simulink model "QEI_READ"  (R2024b)
settings: Solver=FixedStepAuto  StartTime=0.0  StopTime=inf  FixedStep=0.1  RelTol=1e-3  EnableMultiTasking=on
libraries: stm32f4xxblockslib x8, stm32g4xxblockslib x6, simulink x4
settings Model: STM32="{\"EncoderBlockForG4\":[{\"ID\":\"QEI_READ:1\"},{\"ID\":\"QEI_READ:14\"},{\"ID\":\"QEI_READ:15\"},{\"ID\":\"QEI_READ:106\"},{\"ID\":\"QEI_READ:107\"},{\"ID\":\"QEI_READ:108\"}],\"DigitalPortRead\":[{\"ID\":\"QEI_READ:3\"},{\"ID\":\"QEI_READ:4\"},{\"ID\":\"QEI_READ:55\"},{\"ID\":\"QEI_READ:64\"},{\"ID\":\"QEI_READ:78\"},{\"ID\":\"QEI_READ:79\"},{\"ID\":\"QEI_READ:80\"},{\"ID\":\"QEI_READ:81\"}]}"  Creator=asus  LastModifiedBy=asus
settings OptimizationCC: DefaultParameterBehavior=Inlined  EnhancedBackFolding=on  PassReuseOutputArgsAs=Individual arguments  ZeroExternalMemoryAtStartup=off  ZeroInternalMemoryAtStartup=off  MaxStackSize=512  OptimizeBlockOrder=speed  DifferentSizesBufferReuse=on  OptimizationCustomize=off  EfficientTunableParamExpr=on
settings DebuggingCC: ParameterTunabilityLossMsg=error
settings HardwareCC: ProdBitPerPointer=32  ProdBitPerSizeT=32  ProdBitPerPtrDiffT=32  ProdLargestAtomicInteger=Long  ProdLargestAtomicFloat=Double  ProdWordSize=32  ProdLongLongMode=on  ProdHWDeviceType=ARM Compatible->ARM Cortex-M
settings SFSimCC: MATLABDynamicMemAlloc=off
settings RTWCC: Description=Embedded Coder  SystemTargetFile=ert.tlc  HardwareBoard=STM32G4xx Based  TemplateMakefile=ert_default_tmf  Toolchain=GNU Tools for ARM Embedded Processors
settings CodeAppCC: ForceParamTrailComments=on  IgnoreCustomStorageClasses=off  OperatorAnnotations=on  SimulinkDataObjDesc=on  SFDataObjDesc=on  InsertBlockDesc=on
settings ERTTargetCC: TargetLangStandard=C99 (ISO)  CodeReplacementLibrary=ARM Cortex-M  ExtModeTransport=3  ExtModeStaticAlloc=on  ExtModeStaticAllocSize=2048  ExtModeMexFile=ext_xcp  ExtModeIntrfLevel=Level2 - Open

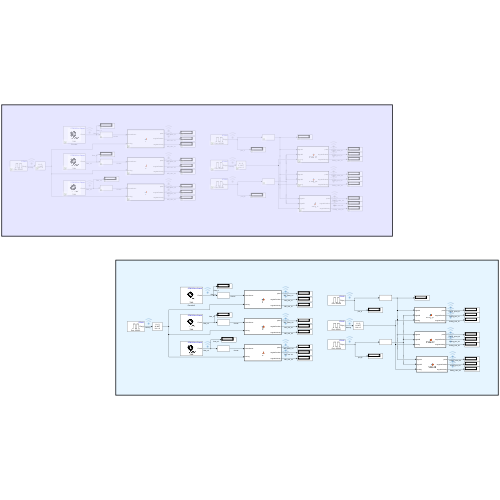
[thumbnail: Simulink's stored preview of the top-level diagram]
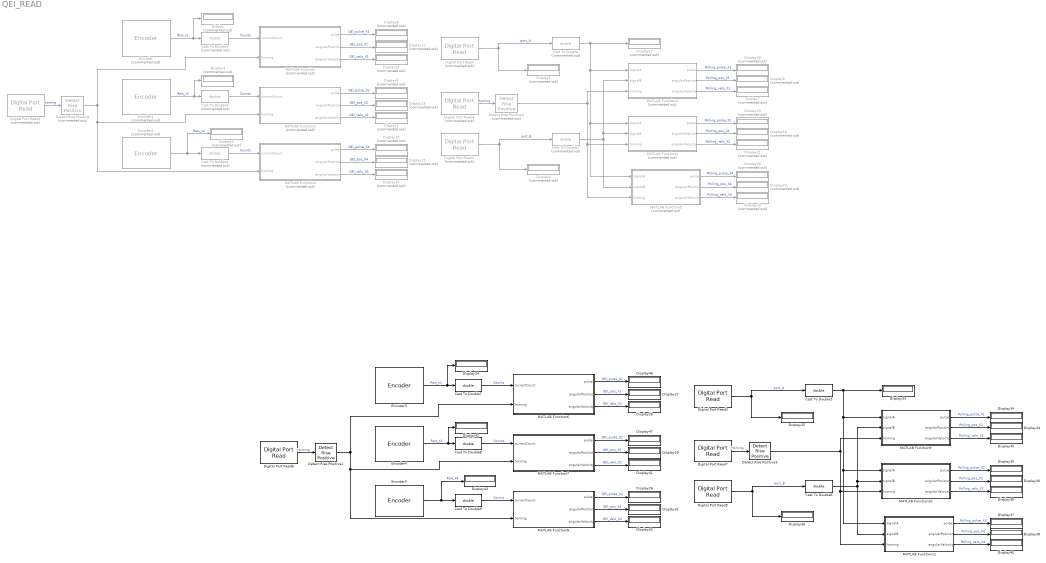
== system QEI_READ ==
  Cast To Double{,1..4} (5 alike) : DataTypeConversion  Commented=on  OutDataTypeStr=double  SaturateOnIntegerOverflow=off  RndMeth=Floor
  Cast To Double{5..9} (5 alike) : DataTypeConversion  OutDataTypeStr=double  SaturateOnIntegerOverflow=off  RndMeth=Floor
  Detect Rise Positive : simulink/Logic and Bit Operations/Detect Rise Positive  Commented=on  vinit=0  OutDataTypeStr=boolean
  Detect Rise Positive1 : simulink/Logic and Bit Operations/Detect Rise Positive  vinit=0  OutDataTypeStr=boolean
  Detect Rise Positive2 : simulink/Logic and Bit Operations/Detect Rise Positive  Commented=on  vinit=0  OutDataTypeStr=boolean
  Detect Rise Positive3 : simulink/Logic and Bit Operations/Detect Rise Positive  vinit=0  OutDataTypeStr=boolean
  Digital Port Read : stm32f4xxblockslib/Digital Port Read  Commented=on  PortName=GPIOB  PinNumber=[10]  ReadOperation=on  IOAsArray=on  SampleTime=-1  EnableSimPort=off  hoistedMaskSrc=ECSoC/ECSimCodegen/Digital Port Read
      settings: LibrarySourceBlock=stm32g4xxblockslib/Digital Port Read
  Digital Port Read1 : stm32f4xxblockslib/Digital Port Read  Commented=on  PortName=GPIOB  PinNumber=[4]  ReadOperation=on  IOAsArray=on  SampleTime=-1  EnableSimPort=off  hoistedMaskSrc=ECSoC/ECSimCodegen/Digital Port Read
      settings: LibrarySourceBlock=stm32g4xxblockslib/Digital Port Read
  Digital Port Read2 : stm32f4xxblockslib/Digital Port Read  Commented=on  PortName=GPIOC  PinNumber=[13]  ReadOperation=on  IOAsArray=on  SampleTime=-1  EnableSimPort=off  hoistedMaskSrc=ECSoC/ECSimCodegen/Digital Port Read
      settings: LibrarySourceBlock=stm32g4xxblockslib/Digital Port Read
  Digital Port Read3 : stm32f4xxblockslib/Digital Port Read  PortName=GPIOB  PinNumber=[10]  ReadOperation=on  IOAsArray=on  SampleTime=-1  EnableSimPort=off  hoistedMaskSrc=ECSoC/ECSimCodegen/Digital Port Read
      settings: LibrarySourceBlock=stm32g4xxblockslib/Digital Port Read
  Digital Port Read4 : stm32f4xxblockslib/Digital Port Read  Commented=on  PortName=GPIOC  PinNumber=[13]  ReadOperation=on  IOAsArray=on  SampleTime=-1  EnableSimPort=off  hoistedMaskSrc=ECSoC/ECSimCodegen/Digital Port Read
      settings: LibrarySourceBlock=stm32g4xxblockslib/Digital Port Read
  Digital Port Read5 : stm32f4xxblockslib/Digital Port Read  PortName=GPIOB  PinNumber=[4]  ReadOperation=on  IOAsArray=on  SampleTime=-1  EnableSimPort=off  hoistedMaskSrc=ECSoC/ECSimCodegen/Digital Port Read
      settings: LibrarySourceBlock=stm32g4xxblockslib/Digital Port Read
  Digital Port Read6 : stm32f4xxblockslib/Digital Port Read  PortName=GPIOC  PinNumber=[13]  ReadOperation=on  IOAsArray=on  SampleTime=-1  EnableSimPort=off  hoistedMaskSrc=ECSoC/ECSimCodegen/Digital Port Read
      settings: LibrarySourceBlock=stm32g4xxblockslib/Digital Port Read
  Digital Port Read7 : stm32f4xxblockslib/Digital Port Read  PortName=GPIOC  PinNumber=[13]  ReadOperation=on  IOAsArray=on  SampleTime=-1  EnableSimPort=off  hoistedMaskSrc=ECSoC/ECSimCodegen/Digital Port Read
      settings: LibrarySourceBlock=stm32g4xxblockslib/Digital Port Read
  Display{,1..23} (24 alike) : Display  Commented=on
  Display{24..47} (24 alike) : Display
  Encoder : stm32g4xxblockslib/Encoder  Commented=on  TimerModule=TIM3  EnableResetInput=off  OutputCountAfterFirstIndex=off  OutputValidIndex=off  OutputDirection=off  OutputStatus=off  SampleTime=-1
  Encoder1 : stm32g4xxblockslib/Encoder  Commented=on  TimerModule=TIM4  EnableResetInput=off  OutputCountAfterFirstIndex=off  OutputValidIndex=off  OutputDirection=off  OutputStatus=off  SampleTime=-1
  Encoder2 : stm32g4xxblockslib/Encoder  Commented=on  TimerModule=TIM8  EnableResetInput=off  OutputCountAfterFirstIndex=off  OutputValidIndex=off  OutputDirection=off  OutputStatus=off  SampleTime=-1
  Encoder3 : stm32g4xxblockslib/Encoder  TimerModule=TIM3  EnableResetInput=off  OutputCountAfterFirstIndex=off  OutputValidIndex=off  OutputDirection=off  OutputStatus=off  SampleTime=-1
  Encoder4 : stm32g4xxblockslib/Encoder  TimerModule=TIM4  EnableResetInput=off  OutputCountAfterFirstIndex=off  OutputValidIndex=off  OutputDirection=off  OutputStatus=off  SampleTime=-1
  Encoder5 : stm32g4xxblockslib/Encoder  TimerModule=TIM8  EnableResetInput=off  OutputCountAfterFirstIndex=off  OutputValidIndex=off  OutputDirection=off  OutputStatus=off  SampleTime=-1
  MATLAB Function : MATLAB Function  Commented=on  TreatAsAtomicUnit=on
  MATLAB Function1 : MATLAB Function  Commented=on  TreatAsAtomicUnit=on
  MATLAB Function10 : MATLAB Function  TreatAsAtomicUnit=on
  MATLAB Function11 : MATLAB Function  TreatAsAtomicUnit=on
  MATLAB Function2 : MATLAB Function  Commented=on  TreatAsAtomicUnit=on
  MATLAB Function3 : MATLAB Function  Commented=on  TreatAsAtomicUnit=on
  MATLAB Function4 : MATLAB Function  Commented=on  TreatAsAtomicUnit=on
  MATLAB Function5 : MATLAB Function  Commented=on  TreatAsAtomicUnit=on
  MATLAB Function6 : MATLAB Function  TreatAsAtomicUnit=on
  MATLAB Function7 : MATLAB Function  TreatAsAtomicUnit=on
  MATLAB Function8 : MATLAB Function  TreatAsAtomicUnit=on
  MATLAB Function9 : MATLAB Function  TreatAsAtomicUnit=on
  wires:
  Encoder/1 -> Display/1, Cast To Double2/1  "Raw_x1"
  Digital Port Read/1 -> Cast To Double/1, Display1/1  "port_A"
  Digital Port Read1/1 -> Cast To Double1/1, Display2/1  "port_B"
  Cast To Double2/1 -> MATLAB Function/1(currentCount)  "Counts"
  MATLAB Function/1(pulse) -> Display8/1  "QEI_pulse_X1"
  MATLAB Function1/1(pulse) -> Display9/1  "QEI_pulse_X2"
  Cast To Double3/1 -> MATLAB Function1/1(currentCount)  "Counts"
  Cast To Double4/1 -> MATLAB Function2/1(currentCount)  "Counts"
  MATLAB Function2/1(pulse) -> Display10/1  "QEI_pulse_X4"
  MATLAB Function/2(angularPosition) -> Display11/1  "QEI_pos_X1"
  MATLAB Function1/2(angularPosition) -> Display13/1  "QEI_pos_X2"
  MATLAB Function2/2(angularPosition) -> Display15/1  "QEI_pos_X4"
  MATLAB Function2/3(angularVelocity) -> Display16/1  "QEI_velo_X4"
  Cast To Double/1 -> Display17/1, MATLAB Function5/1(signalA), MATLAB Function4/1(signalA), MATLAB Function3/1(signalA)
  MATLAB Function3/1(pulse) -> Display18/1  "Polling_pulse_X1"
  MATLAB Function4/1(pulse) -> Display19/1  "Polling_pulse_X2"
  MATLAB Function5/1(pulse) -> Display20/1  "Polling_pulse_X4"
  Cast To Double1/1 -> MATLAB Function4/2(signalB), MATLAB Function3/2(signalB), MATLAB Function5/2(signalB)
  MATLAB Function1/3(angularVelocity) -> Display3/1  "QEI_velo_X2"
  MATLAB Function/3(angularVelocity) -> Display12/1  "QEI_velo_X1"
  Digital Port Read2/1 -> Detect Rise Positive/1  "Homing"
  Detect Rise Positive/1 -> MATLAB Function2/2(homing), MATLAB Function1/2(homing), MATLAB Function/2(homing)
  Encoder1/1 -> Display4/1, Cast To Double3/1  "Raw_x2"
  Encoder2/1 -> Display5/1, Cast To Double4/1  "Raw_x4"
  Digital Port Read4/1 -> Detect Rise Positive2/1  "Homing"
  Detect Rise Positive2/1 -> MATLAB Function5/3(homing), MATLAB Function4/3(homing), MATLAB Function3/3(homing)
  MATLAB Function3/2(angularPosition) -> Display6/1  "Polling_pos_X1"
  MATLAB Function3/3(angularVelocity) -> Display7/1  "Polling_velo_X1"
  MATLAB Function4/2(angularPosition) -> Display14/1  "Polling_pos_X2"
  MATLAB Function4/3(angularVelocity) -> Display21/1  "Polling_velo_X2"
  MATLAB Function5/2(angularPosition) -> Display22/1  "Polling_pos_X4"
  MATLAB Function5/3(angularVelocity) -> Display23/1  "Polling_velo_X4"
  MATLAB Function6/1(pulse) -> Display46/1  "QEI_pulse_X1"
  MATLAB Function7/3(angularVelocity) -> Display41/1  "QEI_velo_X2"
  Digital Port Read5/1 -> Cast To Double6/1, Display36/1  "port_B"
  Cast To Double7/1 -> MATLAB Function6/1(currentCount)  "Counts"
  Digital Port Read6/1 -> Detect Rise Positive1/1  "Homing"
  MATLAB Function7/2(angularPosition) -> Display29/1  "QEI_pos_X2"
  Detect Rise Positive1/1 -> MATLAB Function8/2(homing), MATLAB Function7/2(homing), MATLAB Function6/2(homing)
  Encoder5/1 -> Display43/1, Cast To Double9/1  "Raw_x4"
  Cast To Double6/1 -> MATLAB Function10/2(signalB), MATLAB Function9/2(signalB), MATLAB Function11/2(signalB)
  MATLAB Function9/1(pulse) -> Display34/1  "Polling_pulse_X1"
  MATLAB Function10/3(angularVelocity) -> Display38/1  "Polling_velo_X2"
  MATLAB Function9/3(angularVelocity) -> Display45/1  "Polling_velo_X1"
  MATLAB Function6/2(angularPosition) -> Display27/1  "QEI_pos_X1"
  Digital Port Read3/1 -> Cast To Double5/1, Display25/1  "port_A"
  MATLAB Function8/1(pulse) -> Display26/1  "QEI_pulse_X4"
  Cast To Double5/1 -> Display33/1, MATLAB Function11/1(signalA), MATLAB Function10/1(signalA), MATLAB Function9/1(signalA)
  MATLAB Function9/2(angularPosition) -> Display44/1  "Polling_pos_X1"
  Cast To Double8/1 -> MATLAB Function7/1(currentCount)  "Counts"
  Digital Port Read7/1 -> Detect Rise Positive3/1  "Homing"
  MATLAB Function8/2(angularPosition) -> Display31/1  "QEI_pos_X4"
  Detect Rise Positive3/1 -> MATLAB Function11/3(homing), MATLAB Function10/3(homing), MATLAB Function9/3(homing)
  MATLAB Function11/2(angularPosition) -> Display39/1  "Polling_pos_X4"
  MATLAB Function6/3(angularVelocity) -> Display28/1  "QEI_velo_X1"
  MATLAB Function10/1(pulse) -> Display35/1  "Polling_pulse_X2"
  Encoder3/1 -> Display24/1, Cast To Double7/1  "Raw_x1"
  MATLAB Function11/3(angularVelocity) -> Display40/1  "Polling_velo_X4"
  MATLAB Function7/1(pulse) -> Display47/1  "QEI_pulse_X2"
  MATLAB Function11/1(pulse) -> Display37/1  "Polling_pulse_X4"
  MATLAB Function8/3(angularVelocity) -> Display32/1  "QEI_velo_X4"
  Encoder4/1 -> Display42/1, Cast To Double8/1  "Raw_x2"
  Cast To Double9/1 -> MATLAB Function8/1(currentCount)  "Counts"
  MATLAB Function10/2(angularPosition) -> Display30/1  "Polling_pos_X2"

== matlab function QEI_READ/MATLAB Function6 ==
  data: pulse output; currentCount input; angularPosition output; angularVelocity output; homing input
function [pulse, angularPosition, angularVelocity] = X1(currentCount, homing)
    % พารามิเตอร์ที่ใช้ในการคำนวณ
    maxCount = 65534;           % ค่าสูงสุดที่สามารถนับได้ก่อนจะ wrap-around
    timeInterval = 0.1;         % ช่วงเวลาที่ใช้ในการคำนวณความเร็วเชิงมุม (วินาที)
    PPR = 2048;                   % จำนวนพัลส์ต่อรอบของ Encoder (Pulses Per Revolution)

    % Persistent Variables เพื่อเก็บค่าก่อนหน้า
    persistent previousCount totalCount previousRadians homepos

    % ตั้งค่าเริ่มต้นสำหรับ Persistent Variables
    if isempty(previousCount)
        previousCount = currentCount;
        totalCount = 0;
        previousRadians = 0;
        homepos = 0;
    end

    % คำนวณความแตกต่างระหว่าง currentCount และ previousCount
    diffCount = currentCount - previousCount;

    % ตรวจสอบการเกิด wrap-around
    if diffCount < -maxCount/2
        totalCount = totalCount + (maxCount + diffCount);  % Wrap-around จาก maxCount กลับไปที่ 0
    elseif diffCount > maxCount/2
        totalCount = totalCount + (diffCount - maxCount);  % Wrap-around จาก 0 ไปที่ maxCount
    else
        totalCount = totalCount + diffCount;               % กรณีปกติ ไม่มีการ wrap-around
    end

    % ตั้งค่าโฮม (Home Position) เมื่อ homing == 1
    if homing == 1
        homepos = totalCount;
    end

    % คำนวณตำแหน่งเชิงมุม (Angular Position) และความเร็วเชิงมุม (Angular Velocity)
    pulse = totalCount - homepos;                             % จำนวนพัลส์นับจากตำแหน่งโฮม
    angularPosition = (pulse / PPR) * 2 * pi;                 % แปลงจำนวนพัลส์เป็นตำแหน่งเชิงมุม (radians)
    angularVelocity = (angularPosition - previousRadians) / timeInterval;  % คำนวณความเร็วเชิงมุม

    % อัปเดตค่าก่อนหน้า
    previousCount = currentCount;
    previousRadians = angularPosition;
end

== matlab function QEI_READ/MATLAB Function7 ==
  data: pulse output; currentCount input; angularPosition output; angularVelocity output; homing input
function [pulse, angularPosition, angularVelocity] = X2(currentCount, homing)
    % พารามิเตอร์ที่ใช้ในการคำนวณ
    maxCount = 65534;           % ค่าสูงสุดที่สามารถนับได้ก่อนจะ wrap-around
    timeInterval = 0.1;         % ช่วงเวลาที่ใช้ในการคำนวณความเร็วเชิงมุม (วินาที)
    PPR = 2048;                   % จำนวนพัลส์ต่อรอบของ Encoder (Pulses Per Revolution)

    % Persistent Variables เพื่อเก็บค่าก่อนหน้า
    persistent previousCount totalCount previousRadians homepos

    % ตั้งค่าเริ่มต้นสำหรับ Persistent Variables
    if isempty(previousCount)
        previousCount = currentCount;
        totalCount = 0;
        previousRadians = 0;
        homepos = 0;
    end

    % คำนวณความแตกต่างระหว่าง currentCount และ previousCount
    diffCount = currentCount - previousCount;

    % ตรวจสอบการเกิด wrap-around
    if diffCount < -maxCount/2
        totalCount = totalCount + (maxCount + diffCount);  % Wrap-around จาก maxCount กลับไปที่ 0
    elseif diffCount > maxCount/2
        totalCount = totalCount + (diffCount - maxCount);  % Wrap-around จาก 0 ไปที่ maxCount
    else
        totalCount = totalCount + diffCount;               % กรณีปกติ ไม่มีการ wrap-around
    end

    % ตั้งค่าโฮม (Home Position) เมื่อ homing == 1
    if homing == 1
        homepos = totalCount;
    end

    % คำนวณตำแหน่งเชิงมุม (Angular Position) และความเร็วเชิงมุม (Angular Velocity)
    pulse = totalCount - homepos;                             % จำนวนพัลส์นับจากตำแหน่งโฮม
    angularPosition = (pulse / PPR) * 2 * pi;                 % แปลงจำนวนพัลส์เป็นตำแหน่งเชิงมุม (radians)
    angularVelocity = (angularPosition - previousRadians) / timeInterval;  % คำนวณความเร็วเชิงมุม

    % อัปเดตค่าก่อนหน้า
    previousCount = currentCount;
    previousRadians = angularPosition;
end

== matlab function QEI_READ/MATLAB Function8 ==
  data: pulse output; currentCount input; angularPosition output; angularVelocity output; homing input
function [pulse, angularPosition, angularVelocity] = X4(currentCount, homing)
    % พารามิเตอร์ที่ใช้ในการคำนวณ
    % พารามิเตอร์ที่ใช้ในการคำนวณ
    maxCount = 65534;           % ค่าสูงสุดที่สามารถนับได้ก่อนจะ wrap-around
    timeInterval = 0.1;         % ช่วงเวลาที่ใช้ในการคำนวณความเร็วเชิงมุม (วินาที)
    PPR = 2048;                   % จำนวนพัลส์ต่อรอบของ Encoder (Pulses Per Revolution)

    % Persistent Variables เพื่อเก็บค่าก่อนหน้า
    persistent previousCount totalCount previousRadians homepos

    % ตั้งค่าเริ่มต้นสำหรับ Persistent Variables
    if isempty(previousCount)
        previousCount = currentCount;
        totalCount = 0;
        previousRadians = 0;
        homepos = 0;
    end

    % คำนวณความแตกต่างระหว่าง currentCount และ previousCount
    diffCount = currentCount - previousCount;

    % ตรวจสอบการเกิด wrap-around
    if diffCount < -maxCount/2
        totalCount = totalCount + (maxCount + diffCount);  % Wrap-around จาก maxCount กลับไปที่ 0
    elseif diffCount > maxCount/2
        totalCount = totalCount + (diffCount - maxCount);  % Wrap-around จาก 0 ไปที่ maxCount
    else
        totalCount = totalCount + diffCount;               % กรณีปกติ ไม่มีการ wrap-around
    end

    % ตั้งค่าโฮม (Home Position) เมื่อ homing == 1
    if homing == 1
        homepos = totalCount;
    end

    % คำนวณตำแหน่งเชิงมุม (Angular Position) และความเร็วเชิงมุม (Angular Velocity)
    pulse = totalCount - homepos;                             % จำนวนพัลส์นับจากตำแหน่งโฮม
    angularPosition = (pulse / PPR) * 2 * pi;                 % แปลงจำนวนพัลส์เป็นตำแหน่งเชิงมุม (radians)
    angularVelocity = (angularPosition - previousRadians) / timeInterval;  % คำนวณความเร็วเชิงมุม

    % อัปเดตค่าก่อนหน้า
    previousCount = currentCount;
    previousRadians = angularPosition;
end

== matlab function QEI_READ/MATLAB Function9 ==
  data: signalA input; pulse output; signalB input; homing input; angularPosition output; angularVelocity output
function [pulse, angularPosition, angularVelocity] = Polling_X1(signalA, signalB, homing)
    % กำหนดค่าพารามิเตอร์
    PPR = 2048;               % จำนวนพัลส์ต่อรอบ
    timeInterval = 0.1;     % ช่วงเวลาที่ใช้ในการคำนวณความเร็วเชิงมุม

    % ตัวแปร persistent เพื่อเก็บค่าก่อนหน้าและจำนวนพัลส์ต่อเนื่อง
    persistent previousCount totalCount homepos previousRadians

    % กำหนดค่าเริ่มต้นเมื่อฟังก์ชันถูกเรียกครั้งแรก
    if isempty(previousCount)
        previousCount = 0;
        totalCount = 0;
        homepos = 0;
        previousRadians = 0;
    end

    % คำนวณจำนวนพัลส์ต่อเนื่องตามสัญญาณ A และ B
    if signalA == 1 && signalB == 0
        totalCount = previousCount + 1; % หมุนในทิศทางตามเข็มนาฬิกา
    elseif signalA == 0 && signalB == 1
        totalCount = previousCount - 1; % หมุนในทิศทางตรงกันข้าม
    else
        totalCount = previousCount; % ไม่มีการเปลี่ยนแปลง
    end

% กำหนดตำแหน่งเริ่มต้น (home position) หากอยู่ในโหมด homing
    if homing == 1
        homepos = totalCount;
    end

    % คำนวณค่าพัลส์และตำแหน่งเชิงมุม
    pulse = totalCount - homepos;
    angularPosition = (pulse / PPR) * 2 * pi;

    % คำนวณความเร็วเชิงมุมจากการเปลี่ยนแปลงตำแหน่งเชิงมุมและเวลา
    angularVelocity = (angularPosition - previousRadians) / timeInterval;

    % อัปเดตค่าก่อนหน้าสำหรับรอบถัดไป
    previousCount = totalCount;
    previousRadians = angularPosition;
end

== matlab function QEI_READ/MATLAB Function1 ==
  data: pulse output; currentCount input; angularPosition output; angularVelocity output; homing input
function [pulse, angularPosition, angularVelocity] = X2(currentCount, homing)
    % พารามิเตอร์ที่ใช้ในการคำนวณ
    maxCount = 65520;           % ค่าสูงสุดที่สามารถนับได้ก่อนจะ wrap-around
    timeInterval = 0.1;         % ช่วงเวลาที่ใช้ในการคำนวณความเร็วเชิงมุม (วินาที)
    PPR = 24;                   % จำนวนพัลส์ต่อรอบของ Encoder (Pulses Per Revolution)

    % Persistent Variables เพื่อเก็บค่าก่อนหน้า
    persistent previousCount totalCount previousRadians homepos

    % ตั้งค่าเริ่มต้นสำหรับ Persistent Variables
    if isempty(previousCount)
        previousCount = currentCount;
        totalCount = 0;
        previousRadians = 0;
        homepos = 0;
    end

    % คำนวณความแตกต่างระหว่าง currentCount และ previousCount
    diffCount = currentCount - previousCount;

    % ตรวจสอบการเกิด wrap-around
    if diffCount < -maxCount/2
        totalCount = totalCount + (maxCount + diffCount);  % Wrap-around จาก maxCount กลับไปที่ 0
    elseif diffCount > maxCount/2
        totalCount = totalCount + (diffCount - maxCount);  % Wrap-around จาก 0 ไปที่ maxCount
    else
        totalCount = totalCount + diffCount;               % กรณีปกติ ไม่มีการ wrap-around
    end

    % ตั้งค่าโฮม (Home Position) เมื่อ homing == 1
    if homing == 1
        homepos = totalCount;
    end

    % คำนวณตำแหน่งเชิงมุม (Angular Position) และความเร็วเชิงมุม (Angular Velocity)
    pulse = totalCount - homepos;                             % จำนวนพัลส์นับจากตำแหน่งโฮม
    angularPosition = (pulse / PPR) * 2 * pi;                 % แปลงจำนวนพัลส์เป็นตำแหน่งเชิงมุม (radians)
    angularVelocity = (angularPosition - previousRadians) / timeInterval;  % คำนวณความเร็วเชิงมุม

    % อัปเดตค่าก่อนหน้า
    previousCount = currentCount;
    previousRadians = angularPosition;
end

== matlab function QEI_READ/MATLAB Function ==
  data: pulse output; currentCount input; angularPosition output; angularVelocity output; homing input
function [pulse, angularPosition, angularVelocity] = X1(currentCount, homing)
    % พารามิเตอร์ที่ใช้ในการคำนวณ
    maxCount = 65520;           % ค่าสูงสุดที่สามารถนับได้ก่อนจะ wrap-around
    timeInterval = 0.1;         % ช่วงเวลาที่ใช้ในการคำนวณความเร็วเชิงมุม (วินาที)
    PPR = 24;                   % จำนวนพัลส์ต่อรอบของ Encoder (Pulses Per Revolution)

    % Persistent Variables เพื่อเก็บค่าก่อนหน้า
    persistent previousCount totalCount previousRadians homepos

    % ตั้งค่าเริ่มต้นสำหรับ Persistent Variables
    if isempty(previousCount)
        previousCount = currentCount;
        totalCount = 0;
        previousRadians = 0;
        homepos = 0;
    end

    % คำนวณความแตกต่างระหว่าง currentCount และ previousCount
    diffCount = currentCount - previousCount;

    % ตรวจสอบการเกิด wrap-around
    if diffCount < -maxCount/2
        totalCount = totalCount + (maxCount + diffCount);  % Wrap-around จาก maxCount กลับไปที่ 0
    elseif diffCount > maxCount/2
        totalCount = totalCount + (diffCount - maxCount);  % Wrap-around จาก 0 ไปที่ maxCount
    else
        totalCount = totalCount + diffCount;               % กรณีปกติ ไม่มีการ wrap-around
    end

    % ตั้งค่าโฮม (Home Position) เมื่อ homing == 1
    if homing == 1
        homepos = totalCount;
    end

    % คำนวณตำแหน่งเชิงมุม (Angular Position) และความเร็วเชิงมุม (Angular Velocity)
    pulse = totalCount - homepos;                             % จำนวนพัลส์นับจากตำแหน่งโฮม
    angularPosition = (pulse / PPR) * 2 * pi;                 % แปลงจำนวนพัลส์เป็นตำแหน่งเชิงมุม (radians)
    angularVelocity = (angularPosition - previousRadians) / timeInterval;  % คำนวณความเร็วเชิงมุม

    % อัปเดตค่าก่อนหน้า
    previousCount = currentCount;
    previousRadians = angularPosition;
end

== matlab function QEI_READ/MATLAB Function2 ==
  data: pulse output; currentCount input; angularPosition output; angularVelocity output; homing input
function [pulse, angularPosition, angularVelocity] = X4(currentCount, homing)
    % พารามิเตอร์ที่ใช้ในการคำนวณ
    maxCount = 65520;           % ค่าสูงสุดที่สามารถนับได้ก่อนจะ wrap-around
    timeInterval = 0.1;         % ช่วงเวลาที่ใช้ในการคำนวณความเร็วเชิงมุม (วินาที)
    PPR = 24;                   % จำนวนพัลส์ต่อรอบของ Encoder (Pulses Per Revolution)

    % Persistent Variables เพื่อเก็บค่าก่อนหน้า
    persistent previousCount totalCount previousRadians homepos

    % ตั้งค่าเริ่มต้นสำหรับ Persistent Variables
    if isempty(previousCount)
        previousCount = currentCount;
        totalCount = 0;
        previousRadians = 0;
        homepos = 0;
    end

    % คำนวณความแตกต่างระหว่าง currentCount และ previousCount
    diffCount = currentCount - previousCount;

    % ตรวจสอบการเกิด wrap-around
    if diffCount < -maxCount/2
        totalCount = totalCount + (maxCount + diffCount);  % Wrap-around จาก maxCount กลับไปที่ 0
    elseif diffCount > maxCount/2
        totalCount = totalCount + (diffCount - maxCount);  % Wrap-around จาก 0 ไปที่ maxCount
    else
        totalCount = totalCount + diffCount;               % กรณีปกติ ไม่มีการ wrap-around
    end

    % ตั้งค่าโฮม (Home Position) เมื่อ homing == 1
    if homing == 1
        homepos = totalCount;
    end

    % คำนวณตำแหน่งเชิงมุม (Angular Position) และความเร็วเชิงมุม (Angular Velocity)
    pulse = totalCount - homepos;                             % จำนวนพัลส์นับจากตำแหน่งโฮม
    angularPosition = (pulse / PPR) * 2 * pi;                 % แปลงจำนวนพัลส์เป็นตำแหน่งเชิงมุม (radians)
    angularVelocity = (angularPosition - previousRadians) / timeInterval;  % คำนวณความเร็วเชิงมุม

    % อัปเดตค่าก่อนหน้า
    previousCount = currentCount;
    previousRadians = angularPosition;
end

== matlab function QEI_READ/MATLAB Function3 ==
  data: signalA input; pulse output; signalB input; homing input; angularPosition output; angularVelocity output
function [pulse, angularPosition, angularVelocity] = Polling_X1(signalA, signalB, homing)
    % กำหนดค่าพารามิเตอร์
    PPR = 24;               % จำนวนพัลส์ต่อรอบ
    timeInterval = 0.1;     % ช่วงเวลาที่ใช้ในการคำนวณความเร็วเชิงมุม

    % ตัวแปร persistent เพื่อเก็บค่าก่อนหน้าและจำนวนพัลส์ต่อเนื่อง
    persistent previousCount totalCount homepos previousRadians

    % กำหนดค่าเริ่มต้นเมื่อฟังก์ชันถูกเรียกครั้งแรก
    if isempty(previousCount)
        previousCount = 0;
        totalCount = 0;
        homepos = 0;
        previousRadians = 0;
    end

    % คำนวณจำนวนพัลส์ต่อเนื่องตามสัญญาณ A และ B
    if signalA == 1 && signalB == 0
        totalCount = previousCount + 1; % หมุนในทิศทางตามเข็มนาฬิกา
    elseif signalA == 0 && signalB == 1
        totalCount = previousCount - 1; % หมุนในทิศทางตรงกันข้าม
    else
        totalCount = previousCount; % ไม่มีการเปลี่ยนแปลง
    end

% กำหนดตำแหน่งเริ่มต้น (home position) หากอยู่ในโหมด homing
    if homing == 1
        homepos = totalCount;
    end

    % คำนวณค่าพัลส์และตำแหน่งเชิงมุม
    pulse = totalCount - homepos;
    angularPosition = (pulse / PPR) * 2 * pi;

    % คำนวณความเร็วเชิงมุมจากการเปลี่ยนแปลงตำแหน่งเชิงมุมและเวลา
    angularVelocity = (angularPosition - previousRadians) / timeInterval;

    % อัปเดตค่าก่อนหน้าสำหรับรอบถัดไป
    previousCount = totalCount;
    previousRadians = angularPosition;
end

== matlab function QEI_READ/MATLAB Function4 ==
  data: signalA input; pulse output; signalB input; homing input; angularPosition output; angularVelocity output
function [pulse, angularPosition, angularVelocity] = Polling_X2(signalA, signalB, homing)
    % กำหนดค่าพารามิเตอร์
    PPR = 24;               % จำนวนพัลส์ต่อรอบ
    timeInterval = 0.1;     % ช่วงเวลาที่ใช้ในการคำนวณความเร็วเชิงมุม

    % ตัวแปร persistent เพื่อเก็บค่าก่อนหน้าและจำนวนพัลส์ต่อเนื่อง
    persistent previousCount totalCount homepos previousRadians

    % กำหนดค่าเริ่มต้นเมื่อฟังก์ชันถูกเรียกครั้งแรก
    if isempty(previousCount)
        previousCount = 0;
        totalCount = 0;
        homepos = 0;
        previousRadians = 0;
    end

    % คำนวณจำนวนพัลส์ต่อเนื่องตามสัญญาณ A และ B
    if signalA == 1 && signalB == 0
        totalCount = previousCount + 2; % หมุนในทิศทางตามเข็มนาฬิกา
    elseif signalA == 0 && signalB == 1
        totalCount = previousCount - 2; % หมุนในทิศทางตรงกันข้าม
    else
        totalCount = previousCount; % ไม่มีการเปลี่ยนแปลง
    end

% กำหนดตำแหน่งเริ่มต้น (home position) หากอยู่ในโหมด homing
    if homing == 1
        homepos = totalCount;
    end

    % คำนวณค่าพัลส์และตำแหน่งเชิงมุม
    pulse = totalCount - homepos;
    angularPosition = (pulse / PPR) * 2 * pi;

    % คำนวณความเร็วเชิงมุมจากการเปลี่ยนแปลงตำแหน่งเชิงมุมและเวลา
    angularVelocity = (angularPosition - previousRadians) / timeInterval;

    % อัปเดตค่าก่อนหน้าสำหรับรอบถัดไป
    previousCount = totalCount;
    previousRadians = angularPosition;
end

== matlab function QEI_READ/MATLAB Function5 ==
  data: signalA input; pulse output; signalB input; homing input; angularPosition output; angularVelocity output
function [pulse, angularPosition, angularVelocity] = Polling_X4(signalA, signalB, homing)
    % กำหนดค่าพารามิเตอร์
    PPR = 24;               % จำนวนพัลส์ต่อรอบ
    timeInterval = 0.1;     % ช่วงเวลาที่ใช้ในการคำนวณความเร็วเชิงมุม

    % ตัวแปร persistent เพื่อเก็บค่าก่อนหน้าและจำนวนพัลส์ต่อเนื่อง
    persistent previousCount totalCount homepos previousRadians

    % กำหนดค่าเริ่มต้นเมื่อฟังก์ชันถูกเรียกครั้งแรก
    if isempty(previousCount)
        previousCount = 0;
        totalCount = 0;
        homepos = 0;
        previousRadians = 0;
    end

    % คำนวณจำนวนพัลส์ต่อเนื่องตามสัญญาณ A และ B
    if signalA == 1 && signalB == 0
        totalCount = previousCount + 4; % หมุนในทิศทางตามเข็มนาฬิกา
    elseif signalA == 0 && signalB == 1
        totalCount = previousCount - 4; % หมุนในทิศทางตรงกันข้าม
    else
        totalCount = previousCount; % ไม่มีการเปลี่ยนแปลง
    end

% กำหนดตำแหน่งเริ่มต้น (home position) หากอยู่ในโหมด homing
    if homing == 1
        homepos = totalCount;
    end

    % คำนวณค่าพัลส์และตำแหน่งเชิงมุม
    pulse = totalCount - homepos;
    angularPosition = (pulse / PPR) * 2 * pi;

    % คำนวณความเร็วเชิงมุมจากการเปลี่ยนแปลงตำแหน่งเชิงมุมและเวลา
    angularVelocity = (angularPosition - previousRadians) / timeInterval;

    % อัปเดตค่าก่อนหน้าสำหรับรอบถัดไป
    previousCount = totalCount;
    previousRadians = angularPosition;
end

== matlab function QEI_READ/MATLAB Function10 ==
  data: signalA input; pulse output; signalB input; homing input; angularPosition output; angularVelocity output
function [pulse, angularPosition, angularVelocity] = Polling_X2(signalA, signalB, homing)
    % กำหนดค่าพารามิเตอร์
    PPR = 2048;               % จำนวนพัลส์ต่อรอบ
    timeInterval = 0.1;     % ช่วงเวลาที่ใช้ในการคำนวณความเร็วเชิงมุม

    % ตัวแปร persistent เพื่อเก็บค่าก่อนหน้าและจำนวนพัลส์ต่อเนื่อง
    persistent previousCount totalCount homepos previousRadians

    % กำหนดค่าเริ่มต้นเมื่อฟังก์ชันถูกเรียกครั้งแรก
    if isempty(previousCount)
        previousCount = 0;
        totalCount = 0;
        homepos = 0;
        previousRadians = 0;
    end

    % คำนวณจำนวนพัลส์ต่อเนื่องตามสัญญาณ A และ B
    if signalA == 1 && signalB == 0
        totalCount = previousCount + 2; % หมุนในทิศทางตามเข็มนาฬิกา
    elseif signalA == 0 && signalB == 1
        totalCount = previousCount - 2; % หมุนในทิศทางตรงกันข้าม
    else
        totalCount = previousCount; % ไม่มีการเปลี่ยนแปลง
    end

% กำหนดตำแหน่งเริ่มต้น (home position) หากอยู่ในโหมด homing
    if homing == 1
        homepos = totalCount;
    end

    % คำนวณค่าพัลส์และตำแหน่งเชิงมุม
    pulse = totalCount - homepos;
    angularPosition = (pulse / PPR) * 2 * pi;

    % คำนวณความเร็วเชิงมุมจากการเปลี่ยนแปลงตำแหน่งเชิงมุมและเวลา
    angularVelocity = (angularPosition - previousRadians) / timeInterval;

    % อัปเดตค่าก่อนหน้าสำหรับรอบถัดไป
    previousCount = totalCount;
    previousRadians = angularPosition;
end

== matlab function QEI_READ/MATLAB Function11 ==
  data: signalA input; pulse output; signalB input; homing input; angularPosition output; angularVelocity output
function [pulse, angularPosition, angularVelocity] = Polling_X4(signalA, signalB, homing)
    % กำหนดค่าพารามิเตอร์
    PPR = 2048;               % จำนวนพัลส์ต่อรอบ
    timeInterval = 0.1;     % ช่วงเวลาที่ใช้ในการคำนวณความเร็วเชิงมุม

    % ตัวแปร persistent เพื่อเก็บค่าก่อนหน้าและจำนวนพัลส์ต่อเนื่อง
    persistent previousCount totalCount homepos previousRadians

    % กำหนดค่าเริ่มต้นเมื่อฟังก์ชันถูกเรียกครั้งแรก
    if isempty(previousCount)
        previousCount = 0;
        totalCount = 0;
        homepos = 0;
        previousRadians = 0;
    end

    % คำนวณจำนวนพัลส์ต่อเนื่องตามสัญญาณ A และ B
    if signalA == 1 && signalB == 0
        totalCount = previousCount + 4; % หมุนในทิศทางตามเข็มนาฬิกา
    elseif signalA == 0 && signalB == 1
        totalCount = previousCount - 4; % หมุนในทิศทางตรงกันข้าม
    else
        totalCount = previousCount; % ไม่มีการเปลี่ยนแปลง
    end

% กำหนดตำแหน่งเริ่มต้น (home position) หากอยู่ในโหมด homing
    if homing == 1
        homepos = totalCount;
    end

    % คำนวณค่าพัลส์และตำแหน่งเชิงมุม
    pulse = totalCount - homepos;
    angularPosition = (pulse / PPR) * 2 * pi;

    % คำนวณความเร็วเชิงมุมจากการเปลี่ยนแปลงตำแหน่งเชิงมุมและเวลา
    angularVelocity = (angularPosition - previousRadians) / timeInterval;

    % อัปเดตค่าก่อนหน้าสำหรับรอบถัดไป
    previousCount = totalCount;
    previousRadians = angularPosition;
end
